simulink model "ECS_FOS"  (R2013b)
settings: Solver=ode45  StartTime=0.0  StopTime=10.0  RelTol=1e-3
values from neighbouring files (symbols this model uses):
  FuelBurn = [0 0 0 0 0 0 0 0 0 0 0 0 ... (18249 elements, 1x18249)]    [Benchmark_data1.mat]
undefined symbols (not defined in the file or in its folder): F1, F2, HUGHES_TREITLER, PN_70147
libraries: PowerFlowLib x47, simulink x6
(part 2 of 2)

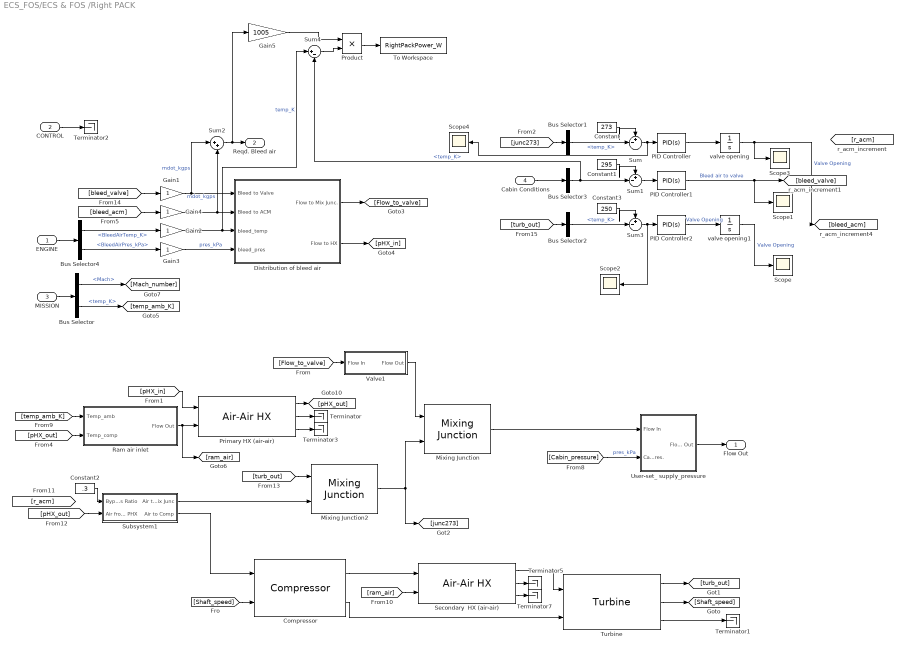
== system ECS_FOS/ECS & FOS /Right PACK ==
  ENGINE : Inport
  CONTROL : Inport  Port=2
  MISSION : Inport  Port=3
  Cabin Conditions : Inport  Port=4
  Bus Selector : BusSelector  OutputSignals=Flight parameters.Mach,Flight parameters.temp_K
  Bus Selector1 : BusSelector  OutputSignals=temp_K
  Bus Selector2 : BusSelector  OutputSignals=temp_K
  Bus Selector3 : BusSelector  OutputSignals=temp_K
  Bus Selector4 : BusSelector  OutputSignals=Bleed.BleedAirTemp_K,Bleed.BleedAirPres_kPa
  Compressor : PowerFlowLib/Energy & Power Systems/Thermal/ECS/Compressor
  Constant : Constant  Value=273
  Constant1 : Constant  Value=295
  Constant2 : Constant  Value=.3
  Constant3 : Constant  Value=250
  Distribution of bleed air : Subsystem
      mask Display:
      | port_label('input',1,'{ \bfBleed air to valve [kg/s]}','texmode','on')
      | port_label('input',2,'{ \bfBleed air to ACM [kg/s]}','texmode','on')
      | port_label('input',3,'{ \bfBleed temp. (K)}','texmode','on');
      | port_label('input',4,'{ \bfBleed pressure. (kPa)}','texmode','on')
      | 
      | 
      | 
      | port_label('output',1,'{\bfFlow to Mix Junc. }','texmode','on')
      | port_label('output',2,'{\bfFlow to ACM }','texmode','on')
  Gain{1..4} (4 alike) : Gain
  Gain5 : Gain  Gain=1005
  Mixing Junction : PowerFlowLib/Energy & Power Systems/Thermal/ECS/Mixing Junction  d_in_1=0.1  d_in_2=0.1  d_out=0.2
  Mixing Junction2 : PowerFlowLib/Energy & Power Systems/Thermal/ECS/Mixing Junction  d_in_1=0.1  d_in_2=0.1  d_out=0.2
  PID Controller : simulink/Continuous/PID Controller  Controller=PID  TimeDomain=Continuous-time  SampleTime=1  IntegratorMethod=Forward Euler  FilterMethod=Forward Euler  Form=Parallel  P=.01  I=0  D=0  N=100  InitialConditionSource=internal  InitialConditionForIntegrator=0  InitialConditionForFilter=0  ExternalReset=none  LimitOutput=off  UpperSaturationLimit=inf  LowerSaturationLimit=-inf  LinearizeAsGain=off  AntiWindupMode=none  Kb=1  TrackingMode=off  Kt=1  PParamMin=[]  PParamMax=[]  IParamMin=[]  IParamMax=[]  DParamMin=[]  DParamMax=[]  NParamMin=[]  NParamMax=[]  KbParamMin=[]  KbParamMax=[]  KtParamMin=[]  KtParamMax=[]  POutMin=[]  POutMax=[]  IOutMin=[]  IOutMax=[]  DOutMin=[]  DOutMax=[]  NOutMin=[]  NOutMax=[]  KbOutMin=[]  KbOutMax=[]  KtOutMin=[]  KtOutMax=[]  IntegratorOutMin=[]  IntegratorOutMax=[]  FilterOutMin=[]  FilterOutMax=[]  SumOutMin=[]  SumOutMax=[]  SumI1OutMin=[]  SumI1OutMax=[]  SumI2OutMin=[]  SumI2OutMax=[]  SumI3OutMin=[]  SumI3OutMax=[]  SumDOutMin=[]  SumDOutMax=[]  SaturationOutMin=[]  SaturationOutMax=[]  IntegratorContinuousStateAttributes=''  IntegratorStateMustResolveToSignalObject=off  IntegratorRTWStateStorageClass=Auto  FilterContinuousStateAttributes=''  FilterStateMustResolveToSignalObject=off  FilterRTWStateStorageClass=Auto
  PID Controller1 : simulink/Continuous/PID Controller  Controller=PID  TimeDomain=Continuous-time  SampleTime=1  IntegratorMethod=Forward Euler  FilterMethod=Forward Euler  Form=Parallel  P=.2  I=.01  D=0  N=100  InitialConditionSource=internal  InitialConditionForIntegrator=0  InitialConditionForFilter=0  ExternalReset=none  LimitOutput=on  UpperSaturationLimit=2  LowerSaturationLimit=.05  LinearizeAsGain=off  AntiWindupMode=none  Kb=1  TrackingMode=off  Kt=1  PParamMin=[]  PParamMax=[]  IParamMin=[]  IParamMax=[]  DParamMin=[]  DParamMax=[]  NParamMin=[]  NParamMax=[]  KbParamMin=[]  KbParamMax=[]  KtParamMin=[]  KtParamMax=[]  POutMin=[]  POutMax=[]  IOutMin=[]  IOutMax=[]  DOutMin=[]  DOutMax=[]  NOutMin=[]  NOutMax=[]  KbOutMin=[]  KbOutMax=[]  KtOutMin=[]  KtOutMax=[]  IntegratorOutMin=[]  IntegratorOutMax=[]  FilterOutMin=[]  FilterOutMax=[]  SumOutMin=[]  SumOutMax=[]  SumI1OutMin=[]  SumI1OutMax=[]  SumI2OutMin=[]  SumI2OutMax=[]  SumI3OutMin=[]  SumI3OutMax=[]  SumDOutMin=[]  SumDOutMax=[]  SaturationOutMin=[]  SaturationOutMax=[]  IntegratorContinuousStateAttributes=''  IntegratorStateMustResolveToSignalObject=off  IntegratorRTWStateStorageClass=Auto  FilterContinuousStateAttributes=''  FilterStateMustResolveToSignalObject=off  FilterRTWStateStorageClass=Auto
  PID Controller2 : simulink/Continuous/PID Controller  Controller=PID  TimeDomain=Continuous-time  SampleTime=1  IntegratorMethod=Forward Euler  FilterMethod=Forward Euler  Form=Parallel  P=0.01  I=0  D=0  N=100  InitialConditionSource=internal  InitialConditionForIntegrator=0  InitialConditionForFilter=0  ExternalReset=none  LimitOutput=off  UpperSaturationLimit=inf  LowerSaturationLimit=0  LinearizeAsGain=off  AntiWindupMode=none  Kb=1  TrackingMode=off  Kt=1  PParamMin=[]  PParamMax=[]  IParamMin=[]  IParamMax=[]  DParamMin=[]  DParamMax=[]  NParamMin=[]  NParamMax=[]  KbParamMin=[]  KbParamMax=[]  KtParamMin=[]  KtParamMax=[]  POutMin=[]  POutMax=[]  IOutMin=[]  IOutMax=[]  DOutMin=[]  DOutMax=[]  NOutMin=[]  NOutMax=[]  KbOutMin=[]  KbOutMax=[]  KtOutMin=[]  KtOutMax=[]  IntegratorOutMin=[]  IntegratorOutMax=[]  FilterOutMin=[]  FilterOutMax=[]  SumOutMin=[]  SumOutMax=[]  SumI1OutMin=[]  SumI1OutMax=[]  SumI2OutMin=[]  SumI2OutMax=[]  SumI3OutMin=[]  SumI3OutMax=[]  SumDOutMin=[]  SumDOutMax=[]  SaturationOutMin=[]  SaturationOutMax=[]  IntegratorContinuousStateAttributes=''  IntegratorStateMustResolveToSignalObject=off  IntegratorRTWStateStorageClass=Auto  FilterContinuousStateAttributes=''  FilterStateMustResolveToSignalObject=off  FilterRTWStateStorageClass=Auto
  Primary HX (air-air) : PowerFlowLib/Energy & Power Systems/Thermal/ECS/Air-Air HX  L_hx=0.2  W_hx=0.2  H_hx=0.2  t_p=0.0008  K_p=167  cp_hx=883  m_cm=16  l_fin=.005  t_fin=0.0002  s_fin=0.0015  h_fin=0.0095  K_n=167  eta_f=0.8  T_cm_0=50
  Product : Product
  Ram air inlet : Subsystem  mask{ram_air=.5, T_35=273}
      mask prompts: ram_air "Ram air mass flow rate"; T_35 "Temperature control for 35F valve"
      mask Display:
      | port_label('input',1,'{ \bf Ambient Temp.}','texmode','on')
      | port_label('input',2,'{ \bf Comp. Face Temp.}','texmode','on');
      | 
      | port_label('output',1,'{\bf Flow Out}','texmode','on')
  Scope{,1..4} (5 alike) : Scope
      Scope settings: SaveName=ScopeData32  SampleInput=on  SampleTime=1
      Scope1 settings: YMin=0  YMax=0.375  SaveName=ScopeData33  SampleInput=on  SampleTime=1
      Scope2 settings: YMin=-0.07  YMax=-0.0325  SaveName=ScopeData34  SampleInput=on  SampleTime=1
      Scope3 settings: YMin=0.427  YMax=0.437  SaveName=ScopeData35  SampleInput=on  SampleTime=1
      Scope4 settings: YMin=0.048825  YMax=0.04905  SaveName=ScopeData37  SampleInput=on  SampleTime=1
  Secondary  HX (air-air) : PowerFlowLib/Energy & Power Systems/Thermal/ECS/Air-Air HX  L_hx=0.2  W_hx=0.2  H_hx=0.2  t_p=0.0008  K_p=167  cp_hx=883  m_cm=16  l_fin=.005  t_fin=0.0002  s_fin=0.0015  h_fin=0.0095  K_n=167  eta_f=0.8  T_cm_0=25
  Subsystem1 : Subsystem
  Sum : Sum  Inputs=+-|
  Sum1 : Sum  Inputs=+-|
  Sum2 : Sum  Inputs=|++
  Sum3 : Sum  Inputs=+-|
  Sum4 : Sum  Inputs=|+-
  Terminator{,1..3,5,7} (6 alike) : Terminator
  To Workspace : ToWorkspace  VariableName=RightPackPower_W  SampleTime=10  SaveFormat=Structure With Time
  Turbine : PowerFlowLib/Energy & Power Systems/Thermal/ECS/Turbine  press_Turbine_exit=80  inertia=5e-5  n_t=0.7
  User-set_ supply_pressure : Subsystem
  Valve1 : Subsystem
  valve opening : Integrator  InitialCondition=.5  LimitOutput=on  UpperSaturationLimit=0.8  LowerSaturationLimit=0.2
  valve opening1 : Integrator  InitialCondition=.5  LimitOutput=on  UpperSaturationLimit=1  LowerSaturationLimit=.3
  Flow Out : Outport
  Reqd. Bleed air : Outport  Port=2
  wires:
  Product/1 -> To Workspace/1
  Sum4/1 -> Product/2
  Gain5/1 -> Product/1
  Sum2/1 -> Reqd. Bleed air/1, Gain5/1
  Gain2/1 -> Distribution of bleed air/3(bleed_temp), Sum4/1  "temp_K"
  Bus Selector3/1 -> Sum1/2, Sum4/2  "<temp_K>"
  Constant2/1 -> Subsystem1/1(Bypass Ratio)
  [bleed_acm] -> Gain4/1
  Constant1/1 -> Sum1/1
  PID Controller1/1 -> [bleed_valve], Scope1/1  "Bleed air to valve"
  Sum1/1 -> PID Controller1/1
  [pHX_in] -> Primary HX (air-air)/1
  Valve1/1(Flow Out) -> Mixing Junction/1
  [Flow_to_valve] -> Valve1/1(Flow In)
  [Shaft_speed] -> Compressor/2
  Compressor/2 -> Turbine/2
  Ram air inlet/1(Flow Out) -> Primary HX (air-air)/2, [ram_air]
  Compressor/1 -> Secondary  HX (air-air)/1
  [ram_air] -> Secondary  HX (air-air)/2
  Mixing Junction/1 -> User-set_ supply_pressure/1(Flow In)
  Turbine/2 -> [Shaft_speed]
  Turbine/3 -> Terminator1/1
  Turbine/1 -> [turb_out]
  User-set_ supply_pressure/1(Flow Out) -> Flow Out/1
  [Cabin_pressure] -> User-set_ supply_pressure/2(Cabin Pres.)  "pres_kPa"
  [temp_amb_K] -> Ram air inlet/1(Temp_amb)
  [pHX_out] -> Ram air inlet/2(Temp_comp)
  MISSION/1 -> Bus Selector/1
  CONTROL/1 -> Terminator2/1
  ENGINE/1 -> Bus Selector4/1
  Distribution of bleed air/2(Flow to HX) -> [pHX_in]
  Distribution of bleed air/1(Flow to Mix Junc.) -> [Flow_to_valve]
  Bus Selector4/1 -> Gain2/1  "<BleedAirTemp_K>"
  Bus Selector4/2 -> Gain3/1  "<BleedAirPres_kPa>"
  Bus Selector/2 -> [temp_amb_K]  "<temp_K>"
  Bus Selector/1 -> [Mach_number]  "<Mach>"
  Gain1/1 -> Distribution of bleed air/1(Bleed to Valve), Sum2/1  "mdot_kgps"
  Gain3/1 -> Distribution of bleed air/4(bleed_pres)  "pres_kPa"
  [bleed_valve] -> Gain1/1
  Primary HX (air-air)/3 -> Terminator3/1
  Primary HX (air-air)/2 -> Terminator/1
  Primary HX (air-air)/1 -> [pHX_out]
  Secondary  HX (air-air)/2 -> Terminator5/1
  Secondary  HX (air-air)/3 -> Terminator7/1
  Secondary  HX (air-air)/1 -> Turbine/1
  [pHX_out] -> Subsystem1/2(Air from PHX)
  Mixing Junction2/1 -> [junc273], Mixing Junction/2
  [turb_out] -> Mixing Junction2/1
  Subsystem1/1(Air to Mix Junc) -> Mixing Junction2/2
  Subsystem1/2(Air to Comp) -> Compressor/1
  [junc273] -> Bus Selector1/1
  Bus Selector1/1 -> Sum/2  "<temp_K>"
  Sum/1 -> PID Controller/1, Scope4/1
  PID Controller/1 -> valve opening/1
  valve opening/1 -> [bleed_acm], Scope3/1  "Valve Opening"
  Constant/1 -> Sum/1
  Gain4/1 -> Distribution of bleed air/2(Bleed to ACM), Sum2/2  "mdot_kgps"
  [turb_out] -> Bus Selector2/1
  Bus Selector2/1 -> Sum3/2  "<temp_K>"
  Sum3/1 -> PID Controller2/1, Scope2/1
  PID Controller2/1 -> valve opening1/1  "Valve Opening"
  Constant3/1 -> Sum3/1
  valve opening1/1 -> Scope/1  "Valve Opening"
  Cabin Conditions/1 -> Bus Selector3/1

== system ECS_FOS/ECS & FOS /Thermal_sources_from Electrical_power_model1 ==
  Gain : Gain
  Terminator : Terminator
  Terminator1 : Terminator
  Terminator2 : Terminator
  ThermalSource : Subsystem  Tag=Flow  Description=TwoPhase  mask(Thermal Source){load_loc=Cockpit}
      mask prompts: load_loc "Location"
      mask help: Output of all thermal loads from the selected location. Loads are in Watts.
      mask init:
      | init_thermal_sourcesink(1)
      settings: CopyFcn=|
      | vals = get_param(gcb,'MaskValues');
      | set_param(gcb,'MaskValues',[vals(1);num2str(0)]);
      mask TypeOptions load_loc: Cockpit | Cabin | CargoBay | LeftWing | RightWing | Empennage
      mask Display:
      | text(.5,.7,'Thermal Source','horizontalAlignment','center','texmode','on')
      | text(.5,.4,get_param(gcb,'load_loc'),'horizontalAlignment','center','texmode','on')
  ThermalSource3 : Subsystem  Tag=Flow  Description=TwoPhase  mask(Thermal Source){load_loc=RightWing}
      mask prompts: load_loc "Location"
      mask help: Output of all thermal loads from the selected location. Loads are in Watts.
      mask init:
      | init_thermal_sourcesink(1)
      settings: CopyFcn=|
      | vals = get_param(gcb,'MaskValues');
      | set_param(gcb,'MaskValues',[vals(1);num2str(0)]);
      mask TypeOptions load_loc: Cockpit | Cabin | CargoBay | LeftWing | RightWing | Empennage
      mask Display:
      | text(.5,.7,'Thermal Source','horizontalAlignment','center','texmode','on')
      | text(.5,.4,get_param(gcb,'load_loc'),'horizontalAlignment','center','texmode','on')
  ThermalSource4 : Subsystem  Tag=Flow  Description=TwoPhase  mask(Thermal Source){load_loc=Empennage}
      mask prompts: load_loc "Location"
      mask help: Output of all thermal loads from the selected location. Loads are in Watts.
      mask init:
      | init_thermal_sourcesink(1)
      settings: CopyFcn=|
      | vals = get_param(gcb,'MaskValues');
      | set_param(gcb,'MaskValues',[vals(1);num2str(0)]);
      mask TypeOptions load_loc: Cockpit | Cabin | CargoBay | LeftWing | RightWing | Empennage
      mask Display:
      | text(.5,.7,'Thermal Source','horizontalAlignment','center','texmode','on')
      | text(.5,.4,get_param(gcb,'load_loc'),'horizontalAlignment','center','texmode','on')
  ThermalSource5 : Subsystem  Tag=Flow  Description=TwoPhase  mask(Thermal Source){load_loc=LeftWing}
      mask prompts: load_loc "Location"
      mask help: Output of all thermal loads from the selected location. Loads are in Watts.
      mask init:
      | init_thermal_sourcesink(1)
      settings: CopyFcn=|
      | vals = get_param(gcb,'MaskValues');
      | set_param(gcb,'MaskValues',[vals(1);num2str(0)]);
      mask TypeOptions load_loc: Cockpit | Cabin | CargoBay | LeftWing | RightWing | Empennage
      mask Display:
      | text(.5,.7,'Thermal Source','horizontalAlignment','center','texmode','on')
      | text(.5,.4,get_param(gcb,'load_loc'),'horizontalAlignment','center','texmode','on')
  Thermal Loads : Outport
  wires:
  ThermalSource5/1(Load) -> Terminator/1
  ThermalSource4/1(Load) -> Terminator2/1
  ThermalSource3/1(Load) -> Terminator1/1
  Gain/1 -> Thermal Loads/1
  ThermalSource/1(Load) -> Gain/1

== system ECS_FOS/Engine #1 - updated 12//1/Heat Loads ==
  Flow In : Inport
  Bus Creator : BusCreator
  Bus Selector : BusSelector  OutputSignals=temp_K,mdot_kgps,pres_kPa,h_kJ/kg
  Gain : Gain  Gain=.1
  Random Number : RandomNumber  Mean=20  Variance=10  SampleTime=0.1
  Sum : Sum  Inputs=++|
  Flow Out : Outport
  wires:
  Flow In/1 -> Bus Selector/1
  Bus Selector/1 -> Sum/2  "<temp_K>"
  Random Number/1 -> Sum/1
  Bus Creator/1 -> Flow Out/1
  Sum/1 -> Bus Creator/1  "temp_K"
  Bus Selector/2 -> Bus Creator/2  "<mdot_kgps>"
  Bus Selector/3 -> Gain/1  "<pres_kPa>"
  Bus Selector/4 -> Bus Creator/4  "<h_kJ/kg>"
  Gain/1 -> Bus Creator/3  "pres_kPa"

== system ECS_FOS/Engine #1 - updated 12//10/Heat Loads ==
  Flow In : Inport
  Bus Creator : BusCreator
  Bus Selector : BusSelector  OutputSignals=temp_K,mdot_kgps,pres_kPa,h_kJ/kg
  Gain : Gain  Gain=.1
  Random Number : RandomNumber  Mean=20  Variance=10  SampleTime=0.1
  Sum : Sum  Inputs=++|
  Flow Out : Outport
  wires:
  Gain/1 -> Bus Creator/3  "pres_kPa"
  Bus Selector/4 -> Bus Creator/4  "<h_kJ/kg>"
  Bus Selector/3 -> Gain/1  "<pres_kPa>"
  Bus Selector/2 -> Bus Creator/2  "<mdot_kgps>"
  Sum/1 -> Bus Creator/1  "temp_K"
  Bus Creator/1 -> Flow Out/1
  Random Number/1 -> Sum/1
  Bus Selector/1 -> Sum/2  "<temp_K>"
  Flow In/1 -> Bus Selector/1

== system ECS_FOS/ECS & FOS /FOHX Left Wing/HX_Calcs ==
  Inputs : Inport
  Bus Creator1 : BusCreator
  Bus Creator2 : BusCreator  Inputs=2
  Fluid 1 Heat Transfer Calculation : Subsystem  TreatAsAtomicUnit=on
  Fluid 2 Heat Transfer Calculation : Subsystem  TreatAsAtomicUnit=on
  Input Processing : Subsystem
  Out : Outport
  wires:
  Fluid 1 Heat Transfer Calculation/3(q_h) -> [q1]
  Fluid 1 Heat Transfer Calculation/2(T_out_h) -> [T1_out]
  Fluid 1 Heat Transfer Calculation/1(h_out_h) -> [h1_out]
  Bus Creator1/1 -> Out/1  "Outputs"
  [Inputs] -> Fluid 1 Heat Transfer Calculation/1(Inputs)
  Inputs/1 -> Input Processing/1(Inputs)  "Inputs"
  Input Processing/1(Processed_Inputs) -> [Inputs]
  Fluid 2 Heat Transfer Calculation/3(q_h) -> [q2]
  Fluid 2 Heat Transfer Calculation/2(T_out) -> [T2_out]
  Fluid 2 Heat Transfer Calculation/1(h_out) -> [h2_out]
  [Inputs] -> Fluid 2 Heat Transfer Calculation/1(Inputs)
  [q1] -> Bus Creator2/1
  [q2] -> Bus Creator2/2
  Bus Creator2/1 -> [q]
  [T2_out] -> Bus Creator1/4  "T2_out"
  [h1_out] -> Bus Creator1/1  "h1_out"
  [T1_out] -> Bus Creator1/2  "T1_out"
  [h2_out] -> Bus Creator1/3  "h2_out"

== system ECS_FOS/ECS & FOS /FOHX Right Wing/HX_Calcs ==
  Inputs : Inport
  Bus Creator1 : BusCreator
  Bus Creator2 : BusCreator  Inputs=2
  Fluid 1 Heat Transfer Calculation : Subsystem  TreatAsAtomicUnit=on
  Fluid 2 Heat Transfer Calculation : Subsystem  TreatAsAtomicUnit=on
  Input Processing : Subsystem
  Out : Outport
  wires:
  [h2_out] -> Bus Creator1/3  "h2_out"
  [T1_out] -> Bus Creator1/2  "T1_out"
  [h1_out] -> Bus Creator1/1  "h1_out"
  [T2_out] -> Bus Creator1/4  "T2_out"
  Bus Creator2/1 -> [q]
  [q2] -> Bus Creator2/2
  [q1] -> Bus Creator2/1
  [Inputs] -> Fluid 2 Heat Transfer Calculation/1(Inputs)
  Fluid 2 Heat Transfer Calculation/1(h_out) -> [h2_out]
  Fluid 2 Heat Transfer Calculation/2(T_out) -> [T2_out]
  Fluid 2 Heat Transfer Calculation/3(q_h) -> [q2]
  Input Processing/1(Processed_Inputs) -> [Inputs]
  Inputs/1 -> Input Processing/1(Inputs)  "Inputs"
  [Inputs] -> Fluid 1 Heat Transfer Calculation/1(Inputs)
  Bus Creator1/1 -> Out/1  "Outputs"
  Fluid 1 Heat Transfer Calculation/1(h_out_h) -> [h1_out]
  Fluid 1 Heat Transfer Calculation/2(T_out_h) -> [T1_out]
  Fluid 1 Heat Transfer Calculation/3(q_h) -> [q1]

== system ECS_FOS/ECS & FOS /Fuel Tanks//Pumps/FlowGenerator1 ==
  Bias : Bias  Bias=273.15
  Bus Creator1 : BusCreator
  Constant3 : Constant  Value=flowenthalpy
  Constant5 : Constant  Value=flowrate
  Constant6 : Constant  Value=flowtemp
  Constant7 : Constant  Value=flowpres
  FlowOut : Outport  Tag=Flow Out
  wires:
  Bus Creator1/1 -> FlowOut/1  "Outlet"
  Constant6/1 -> Bias/1  "temp_C"
  Constant7/1 -> Bus Creator1/3  "pres_kPa"
  Constant3/1 -> Bus Creator1/4  "H_kJpkg"
  Constant5/1 -> Bus Creator1/1  "mdot_kgps"
  Bias/1 -> Bus Creator1/2  "temp_K"

== system ECS_FOS/ECS & FOS /Fuel Tanks//Pumps/Fuel Control Left Wing ==
  FuelNeed : Inport
  FuelFromPump : Inport  Port=2
  Bus Creator : BusCreator  Inputs=3
  Bus Creator1 : BusCreator  Inputs=3
  Bus Selector : BusSelector  OutputSignals=mdot_kgps,temp_K,pres_kPa
  Gain : Gain
  Gain1 : Gain
  Saturation : Saturate  UpperLimit=inf  LowerLimit=0
  Sum : Sum  Inputs=|+-
  Switch : Switch  Criteria=u2 > Threshold
  Fuel2Engine : Outport
  Fuel2Tank : Outport  Port=2
  wires:
  FuelFromPump/1 -> Bus Selector/1
  Bus Selector/1 -> Sum/1, Switch/3  "<mdot_kgps>"
  FuelNeed/1 -> Sum/2, Switch/1
  Sum/1 -> Saturation/1, Switch/2
  Bus Creator/1 -> Fuel2Tank/1
  Bus Selector/2 -> Bus Creator/2, Gain1/1  "<temp_K>"
  Saturation/1 -> Bus Creator/1  "mdot_kgps"
  Switch/1 -> Bus Creator1/1  "mdot_kgps"
  Bus Selector/3 -> Bus Creator/3, Gain/1  "<pres_kPa>"
  Bus Creator1/1 -> Fuel2Engine/1
  Gain/1 -> Bus Creator1/3  "pres_kPa"
  Gain1/1 -> Bus Creator1/2  "temp_K"

== system ECS_FOS/ECS & FOS /Fuel Tanks//Pumps/Fuel Control Right Wing  ==
  FuelNeed : Inport
  FuelFromPump : Inport  Port=2
  Bus Creator : BusCreator  Inputs=3
  Bus Creator1 : BusCreator  Inputs=3
  Bus Selector : BusSelector  OutputSignals=mdot_kgps,temp_K,pres_kPa
  Gain : Gain
  Gain1 : Gain
  Saturation : Saturate  UpperLimit=inf  LowerLimit=0
  Sum : Sum  Inputs=|+-
  Switch : Switch  Criteria=u2 > Threshold
  Fuel2Engine : Outport
  Fuel2Tank : Outport  Port=2
  wires:
  Gain1/1 -> Bus Creator1/2  "temp_K"
  Gain/1 -> Bus Creator1/3  "pres_kPa"
  Bus Creator1/1 -> Fuel2Engine/1
  Bus Selector/3 -> Gain/1, Bus Creator/3  "<pres_kPa>"
  Switch/1 -> Bus Creator1/1  "mdot_kgps"
  Saturation/1 -> Bus Creator/1  "mdot_kgps"
  Bus Selector/2 -> Gain1/1, Bus Creator/2  "<temp_K>"
  Bus Creator/1 -> Fuel2Tank/1
  Sum/1 -> Switch/2, Saturation/1
  FuelNeed/1 -> Switch/1, Sum/2
  Bus Selector/1 -> Switch/3, Sum/1  "<mdot_kgps>"
  FuelFromPump/1 -> Bus Selector/1

== system ECS_FOS/ECS & FOS /Fuel Tanks//Pumps/Fuel Switch On//Off ==
  Right Wing Tank : Inport
  Center Tank : Inport  Port=2
  Left Wing Tank : Inport  Port=3
  Operating RPM : Constant  Value=6000
  Operating RPM1 : Constant  Value=6000
  Operating RPM2 : Constant  Value=6000
  Right Wing Fuel Pumps On/Off : Switch  Criteria=u2 ~= 0
  Right Wing Fuel Pumps On/Off1 : Switch  Criteria=u2 ~= 0
  Right Wing Fuel Pumps On/Off2 : Switch  Criteria=u2 ~= 0
  shut off : Constant  Value=0
  shut off1 : Constant  Value=0
  shut off2 : Constant  Value=0
  Right Wing RPM : Outport
  Left Wing RPM : Outport  Port=2
  Center RPM : Outport  Port=3
  wires:
  Right Wing Fuel Pumps On/Off2/1 -> Left Wing RPM/1
  Right Wing Fuel Pumps On/Off1/1 -> Center RPM/1
  Right Wing Fuel Pumps On/Off/1 -> Right Wing RPM/1
  Left Wing Tank/1 -> Right Wing Fuel Pumps On/Off2/2
  shut off2/1 -> Right Wing Fuel Pumps On/Off2/3
  Operating RPM2/1 -> Right Wing Fuel Pumps On/Off2/1
  Center Tank/1 -> Right Wing Fuel Pumps On/Off1/2
  shut off1/1 -> Right Wing Fuel Pumps On/Off1/3
  Operating RPM1/1 -> Right Wing Fuel Pumps On/Off1/1
  Right Wing Tank/1 -> Right Wing Fuel Pumps On/Off/2
  shut off/1 -> Right Wing Fuel Pumps On/Off/3
  Operating RPM/1 -> Right Wing Fuel Pumps On/Off/1

== system ECS_FOS/ECS & FOS /Fuel Tanks//Pumps/Pump Split ==
  Flow In : Inport
  Bus Creator : BusCreator
  Bus Selector14 : BusSelector  OutputSignals=temp_K,mdot_kgps,pres_kPa,H_kJpkg
  Gain : Gain  Gain=0.5
  Flow Out : Outport
  wires:
  Flow In/1 -> Bus Selector14/1
  Bus Selector14/2 -> Gain/1  "<mdot_kgps>"
  Bus Creator/1 -> Flow Out/1
  Bus Selector14/1 -> Bus Creator/1  "<temp_K>"
  Gain/1 -> Bus Creator/2  "mdot_kgps"
  Bus Selector14/3 -> Bus Creator/3  "<pres_kPa>"
  Bus Selector14/4 -> Bus Creator/4  "<H_kJpkg>"

== system ECS_FOS/ECS & FOS /Fuel Tanks//Pumps/Pump Split1 ==
  Flow In : Inport
  Bus Creator : BusCreator
  Bus Selector14 : BusSelector  OutputSignals=temp_K,mdot_kgps,pres_kPa,H_kJpkg
  Gain : Gain  Gain=0.5
  Flow Out : Outport
  wires:
  Bus Selector14/4 -> Bus Creator/4  "<H_kJpkg>"
  Bus Selector14/3 -> Bus Creator/3  "<pres_kPa>"
  Gain/1 -> Bus Creator/2  "mdot_kgps"
  Bus Selector14/1 -> Bus Creator/1  "<temp_K>"
  Bus Creator/1 -> Flow Out/1
  Bus Selector14/2 -> Gain/1  "<mdot_kgps>"
  Flow In/1 -> Bus Selector14/1

== system ECS_FOS/ECS & FOS /Fuel Tanks//Pumps/Pump Split2 ==
  Flow In : Inport
  Bus Creator : BusCreator
  Bus Selector14 : BusSelector  OutputSignals=temp_K,mdot_kgps,pres_kPa,H_kJpkg
  Gain : Gain  Gain=0.5
  Flow Out : Outport
  wires:
  Bus Selector14/4 -> Bus Creator/4  "<H_kJpkg>"
  Bus Selector14/3 -> Bus Creator/3  "<pres_kPa>"
  Gain/1 -> Bus Creator/2  "mdot_kgps"
  Bus Selector14/1 -> Bus Creator/1  "<temp_K>"
  Bus Creator/1 -> Flow Out/1
  Bus Selector14/2 -> Gain/1  "<mdot_kgps>"
  Flow In/1 -> Bus Selector14/1

== system ECS_FOS/ECS & FOS /Left PACK/Distribution of bleed air ==
  Bleed to Valve : Inport
  Bleed to ACM : Inport  Port=2
  bleed_temp : Inport  Port=3
  bleed_pres : Inport  Port=4
  Bus Creator1 : BusCreator  Inputs=3
  Bus Creator2 : BusCreator  Inputs=3
  Scope : Scope  NumInputPorts=4
      settings: YMin=0~386.7~110~0.2  YMax=0.055~387.8~160~0.85  SaveName=ScopeData42  SampleInput=on  SampleTime=1
  Flow to Mix Junc. : Outport
  Flow to HX : Outport  Port=2
  wires:
  Bus Creator2/1 -> Flow to HX/1
  Bus Creator1/1 -> Flow to Mix Junc./1
  Bleed to Valve/1 -> Scope/1, Bus Creator1/1  "mdot_kgps"
  bleed_pres/1 -> Scope/3, Bus Creator1/3, Bus Creator2/3
  bleed_temp/1 -> Scope/2, Bus Creator1/2, Bus Creator2/2
  Bleed to ACM/1 -> Scope/4, Bus Creator2/1  "mdot_kgps"

== system ECS_FOS/ECS & FOS /Left PACK/Ram air inlet ==
  Temp_amb : Inport
  Temp_comp : Inport  Port=2
  2 : Constant  Value=T_35
  Bus Creator : BusCreator  Inputs=3
  Bus Selector4 : BusSelector  OutputSignals=temp_K
  Constant1 : Constant  Value=22.5
  Gain : Gain  Gain=0.95
  Gain1 : Gain
  Memory : Memory  X0=ram_air
  Subtract : Sum  Inputs=+-
  Switch : Switch  Criteria=u2 ~= 0  Threshold=30
  Flow Out : Outport
  wires:
  Gain1/1 -> Switch/1
  Memory/1 -> Gain/1, Gain1/1, Bus Creator/3  "mdot_kgps"
  Bus Creator/1 -> Flow Out/1
  Constant1/1 -> Bus Creator/2  "pres_kPa"
  Temp_amb/1 -> Bus Creator/1  "temp_K"
  Switch/1 -> Memory/1
  Gain/1 -> Switch/3
  Subtract/1 -> Switch/2
  2/1 -> Subtract/2
  Bus Selector4/1 -> Subtract/1  "<temp_K>"
  Temp_comp/1 -> Bus Selector4/1

== system ECS_FOS/ECS & FOS /Left PACK/Subsystem1 ==
  Bypass Ratio : Inport
  Air from PHX : Inport  Port=2
  Bus Creator : BusCreator  Inputs=3
  Bus Creator1 : BusCreator  Inputs=3
  Bus Selector : BusSelector  OutputSignals=mdot_kgps,temp_K,pres_kPa
  Fcn1 : Fcn  Expr=1-u(1)
  Gain : Gain
  Gain1 : Gain
  Gain2 : Gain
  Product : Product  RndMeth=Zero
  Product1 : Product  RndMeth=Zero
  Saturation : Saturate  UpperLimit=inf  LowerLimit=eps
  Air to Mix Junc : Outport
  Air to Comp : Outport  Port=2
  wires:
  Gain2/1 -> Bus Creator/3  "pres_kPa"
  Fcn1/1 -> Product/1
  Bypass Ratio/1 -> Product1/2, Fcn1/1
  Product/1 -> Saturation/1
  Air from PHX/1 -> Bus Selector/1
  Bus Selector/1 -> Product1/1, Product/2  "<mdot_kgps>"
  Bus Creator/1 -> Air to Comp/1
  Bus Selector/2 -> Bus Creator/2, Gain1/1  "<temp_K>"
  Saturation/1 -> Bus Creator/1  "mdot_kgps"
  Product1/1 -> Bus Creator1/1  "mdot_kgps"
  Bus Selector/3 -> Gain2/1, Gain/1  "<pres_kPa>"
  Bus Creator1/1 -> Air to Mix Junc/1
  Gain/1 -> Bus Creator1/3  "pres_kPa"
  Gain1/1 -> Bus Creator1/2  "temp_K"

== system ECS_FOS/ECS & FOS /Left PACK/User-set_ supply_pressure ==
  Flow In : Inport
  Cabin Pres. : Inport  Port=2
  Bus Creator4 : BusCreator  Inputs=3
  Bus Selector3 : BusSelector  OutputSignals=mdot_kgps,temp_K
  Gain1 : Gain  Gain=1.1
  Flow Out : Outport
  wires:
  Cabin Pres./1 -> Gain1/1
  Bus Creator4/1 -> Flow Out/1
  Flow In/1 -> Bus Selector3/1
  Gain1/1 -> Bus Creator4/3  "pres_kPa"
  Bus Selector3/2 -> Bus Creator4/2  "<temp_K>"
  Bus Selector3/1 -> Bus Creator4/1  "<mdot_kgps>"

== system ECS_FOS/ECS & FOS /Left PACK/Valve1 ==
  Flow In : Inport
  Bus Creator2 : BusCreator  Inputs=3
  Bus Selector2 : BusSelector  OutputSignals=mdot_kgps,pres_kPa,temp_K
  Math Functin : Math  Operator=pow  SaturateOnIntegerOverflow=on
  Product : Product  RndMeth=Zero
  Sum : Sum  Inputs=|-+
  "Value?? -- MAW" : Constant  Value=50
  get u : Gain
  mass_flow_rate1 : Constant  Value=2
  Flow Out : Outport
  wires:
  "Value?? -- MAW"/1 -> Product/1
  Bus Selector2/3 -> Bus Creator2/3  "<temp_K>"
  Sum/1 -> Bus Creator2/2  "pres_kPa"
  Bus Selector2/2 -> Sum/2  "<pres_kPa>"
  Product/1 -> Sum/1
  Math Functin/1 -> Product/2
  mass_flow_rate1/1 -> Math Functin/2
  get u/1 -> Math Functin/1
  Bus Selector2/1 -> get u/1, Bus Creator2/1  "<mdot_kgps>"
  Flow In/1 -> Bus Selector2/1
  Bus Creator2/1 -> Flow Out/1

== system ECS_FOS/ECS & FOS /Right PACK/Distribution of bleed air ==
  Bleed to Valve : Inport
  Bleed to ACM : Inport  Port=2
  bleed_temp : Inport  Port=3
  bleed_pres : Inport  Port=4
  Bus Creator1 : BusCreator  Inputs=3
  Bus Creator2 : BusCreator  Inputs=3
  Scope : Scope  NumInputPorts=4
      settings: YMin=0~386.7~110~0.2  YMax=0.055~387.8~160~0.85  SaveName=ScopeData42  SampleInput=on  SampleTime=1
  Flow to Mix Junc. : Outport
  Flow to HX : Outport  Port=2
  wires:
  Bleed to ACM/1 -> Bus Creator2/1, Scope/4  "mdot_kgps"
  bleed_temp/1 -> Bus Creator2/2, Bus Creator1/2, Scope/2
  bleed_pres/1 -> Bus Creator2/3, Bus Creator1/3, Scope/3
  Bleed to Valve/1 -> Bus Creator1/1, Scope/1  "mdot_kgps"
  Bus Creator1/1 -> Flow to Mix Junc./1
  Bus Creator2/1 -> Flow to HX/1

== system ECS_FOS/ECS & FOS /Right PACK/Ram air inlet ==
  Temp_amb : Inport
  Temp_comp : Inport  Port=2
  2 : Constant  Value=T_35
  Bus Creator : BusCreator  Inputs=3
  Bus Selector4 : BusSelector  OutputSignals=temp_K
  Constant1 : Constant  Value=22.5
  Gain : Gain  Gain=0.95
  Gain1 : Gain
  Memory : Memory  X0=ram_air
  Subtract : Sum  Inputs=+-
  Switch : Switch  Criteria=u2 ~= 0  Threshold=30
  Flow Out : Outport
  wires:
  Temp_comp/1 -> Bus Selector4/1
  Bus Selector4/1 -> Subtract/1  "<temp_K>"
  2/1 -> Subtract/2
  Subtract/1 -> Switch/2
  Gain/1 -> Switch/3
  Switch/1 -> Memory/1
  Temp_amb/1 -> Bus Creator/1  "temp_K"
  Constant1/1 -> Bus Creator/2  "pres_kPa"
  Bus Creator/1 -> Flow Out/1
  Memory/1 -> Bus Creator/3, Gain1/1, Gain/1  "mdot_kgps"
  Gain1/1 -> Switch/1

== system ECS_FOS/ECS & FOS /Right PACK/Subsystem1 ==
  Bypass Ratio : Inport
  Air from PHX : Inport  Port=2
  Bus Creator : BusCreator  Inputs=3
  Bus Creator1 : BusCreator  Inputs=3
  Bus Selector : BusSelector  OutputSignals=mdot_kgps,temp_K,pres_kPa
  Fcn1 : Fcn  Expr=1-u(1)
  Gain : Gain
  Gain1 : Gain
  Gain2 : Gain
  Product : Product  RndMeth=Zero
  Product1 : Product  RndMeth=Zero
  Saturation : Saturate  UpperLimit=inf  LowerLimit=eps
  Air to Mix Junc : Outport
  Air to Comp : Outport  Port=2
  wires:
  Gain1/1 -> Bus Creator1/2  "temp_K"
  Gain/1 -> Bus Creator1/3  "pres_kPa"
  Bus Creator1/1 -> Air to Mix Junc/1
  Bus Selector/3 -> Gain/1, Gain2/1  "<pres_kPa>"
  Product1/1 -> Bus Creator1/1  "mdot_kgps"
  Saturation/1 -> Bus Creator/1  "mdot_kgps"
  Bus Selector/2 -> Gain1/1, Bus Creator/2  "<temp_K>"
  Bus Creator/1 -> Air to Comp/1
  Bus Selector/1 -> Product/2, Product1/1  "<mdot_kgps>"
  Air from PHX/1 -> Bus Selector/1
  Product/1 -> Saturation/1
  Bypass Ratio/1 -> Fcn1/1, Product1/2
  Fcn1/1 -> Product/1
  Gain2/1 -> Bus Creator/3  "pres_kPa"

== system ECS_FOS/ECS & FOS /Right PACK/User-set_ supply_pressure ==
  Flow In : Inport
  Cabin Pres. : Inport  Port=2
  Bus Creator4 : BusCreator  Inputs=3
  Bus Selector3 : BusSelector  OutputSignals=mdot_kgps,temp_K
  Gain1 : Gain  Gain=1.1
  Flow Out : Outport
  wires:
  Bus Selector3/1 -> Bus Creator4/1  "<mdot_kgps>"
  Bus Selector3/2 -> Bus Creator4/2  "<temp_K>"
  Gain1/1 -> Bus Creator4/3  "pres_kPa"
  Flow In/1 -> Bus Selector3/1
  Bus Creator4/1 -> Flow Out/1
  Cabin Pres./1 -> Gain1/1

== system ECS_FOS/ECS & FOS /Right PACK/Valve1 ==
  Flow In : Inport
  Bus Creator2 : BusCreator  Inputs=3
  Bus Selector2 : BusSelector  OutputSignals=mdot_kgps,pres_kPa,temp_K
  Math Functin : Math  Operator=pow  SaturateOnIntegerOverflow=on
  Product : Product  RndMeth=Zero
  Sum : Sum  Inputs=|-+
  "Value?? -- MAW" : Constant  Value=50
  get u : Gain
  mass_flow_rate1 : Constant  Value=2
  Flow Out : Outport
  wires:
  Bus Creator2/1 -> Flow Out/1
  Flow In/1 -> Bus Selector2/1
  Bus Selector2/1 -> Bus Creator2/1, get u/1  "<mdot_kgps>"
  get u/1 -> Math Functin/1
  mass_flow_rate1/1 -> Math Functin/2
  Math Functin/1 -> Product/2
  Product/1 -> Sum/1
  Bus Selector2/2 -> Sum/2  "<pres_kPa>"
  Sum/1 -> Bus Creator2/2  "pres_kPa"
  Bus Selector2/3 -> Bus Creator2/3  "<temp_K>"
  "Value?? -- MAW"/1 -> Product/1

== system ECS_FOS/ECS & FOS /Thermal_sources_from Electrical_power_model1/ThermalSource ==
  LoadBus : BusCreator  Inputs=1
  Load : Outport
  wires:
  LoadBus/1 -> Load/1

== system ECS_FOS/ECS & FOS /Thermal_sources_from Electrical_power_model1/ThermalSource3 ==
  LoadBus : BusCreator  Inputs=1
  Load : Outport
  wires:
  LoadBus/1 -> Load/1

== system ECS_FOS/ECS & FOS /Thermal_sources_from Electrical_power_model1/ThermalSource4 ==
  LoadBus : BusCreator  Inputs=1
  Load : Outport
  wires:
  LoadBus/1 -> Load/1

== system ECS_FOS/ECS & FOS /Thermal_sources_from Electrical_power_model1/ThermalSource5 ==
  LoadBus : BusCreator  Inputs=1
  Load : Outport
  wires:
  LoadBus/1 -> Load/1

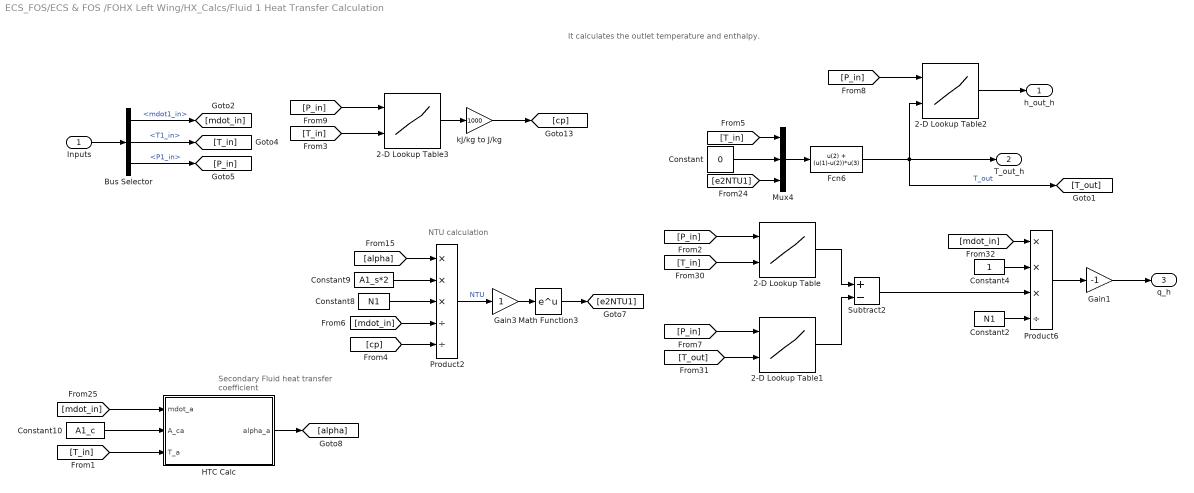
== system ECS_FOS/ECS & FOS /FOHX Left Wing/HX_Calcs/Fluid 1 Heat Transfer Calculation ==
  note: NTU calculation
  note: Secondary Fluid heat transfer coefficient
  note: It calculates the outlet temperature and enthalpy.
  Inputs : Inport
  2-D Lookup Table : Lookup_n-D  BreakpointsForDimension1=F1.P  BreakpointsForDimension2=F1.T  Table=F1.H_pt  RndMeth=Simplest  InputSameDT=on
  2-D Lookup Table1 : Lookup_n-D  BreakpointsForDimension1=F1.P  BreakpointsForDimension2=F1.T  Table=F1.H_pt  RndMeth=Simplest  InputSameDT=on
  2-D Lookup Table2 : Lookup_n-D  BreakpointsForDimension1=F1.P  BreakpointsForDimension2=F1.T  Table=F1.H_pt  RndMeth=Simplest  InputSameDT=on
  2-D Lookup Table3 : Lookup_n-D  BreakpointsForDimension1=F1.P  BreakpointsForDimension2=F1.T  Table=F1.Cp_pt  RndMeth=Simplest  InputSameDT=on
  Bus Selector : BusSelector  OutputSignals=mdot1_in,T1_in,P1_in
  Constant : Constant  Value=0
  Constant10 : Constant  Value=A1_c
  Constant2 : Constant  Value=N1
  Constant4 : Constant
  Constant8 : Constant  Value=N1
  Constant9 : Constant  Value=A1_s*2
  Fcn6 : Fcn  Expr=u(2) + (u(1)-u(2))*u(3)
  Gain1 : Gain  Gain=-1
  Gain3 : Gain
  HTC Calc : Subsystem
  Math Function3 : Math  SaturateOnIntegerOverflow=on
  Mux4 : Mux  Inputs=3
  Product2 : Product  Inputs=***//  RndMeth=Zero
  Product6 : Product  Inputs=***/  RndMeth=Zero
  Subtract2 : Sum  Inputs=+-
  kJ/kg to J/kg : Gain  Gain=1000
  h_out_h : Outport
  T_out_h : Outport  Port=2
  q_h : Outport  Port=3
  wires:
  [T_out] -> 2-D Lookup Table1/2
  [T_in] -> 2-D Lookup Table/2
  2-D Lookup Table/1 -> Subtract2/1
  2-D Lookup Table1/1 -> Subtract2/2
  2-D Lookup Table2/1 -> h_out_h/1
  Product6/1 -> Gain1/1
  Constant4/1 -> Product6/2
  [mdot_in] -> Product6/1
  Subtract2/1 -> Product6/3
  Fcn6/1 -> T_out_h/1, [T_out], 2-D Lookup Table2/2  "T_out"
  Mux4/1 -> Fcn6/1
  [e2NTU1] -> Mux4/3
  Constant/1 -> Mux4/2
  Gain1/1 -> q_h/1
  Constant2/1 -> Product6/4
  Product2/1 -> Gain3/1  "NTU"
  Constant9/1 -> Product2/2
  [alpha] -> Product2/1
  Constant8/1 -> Product2/3
  HTC Calc/1(alpha_a) -> [alpha]
  [T_in] -> HTC Calc/3(T_a)
  Constant10/1 -> HTC Calc/2(A_ca)
  [mdot_in] -> HTC Calc/1(mdot_a)
  [T_in] -> 2-D Lookup Table3/2
  2-D Lookup Table3/1 -> kJ/kg to J/kg/1
  Inputs/1 -> Bus Selector/1
  Bus Selector/1 -> [mdot_in]  "<mdot1_in>"
  Bus Selector/2 -> [T_in]  "<T1_in>"
  Bus Selector/3 -> [P_in]  "<P1_in>"
  Math Function3/1 -> [e2NTU1]
  Gain3/1 -> Math Function3/1
  [mdot_in] -> Product2/4
  [cp] -> Product2/5
  [T_in] -> Mux4/1
  [P_in] -> 2-D Lookup Table/1
  [P_in] -> 2-D Lookup Table1/1
  [P_in] -> 2-D Lookup Table2/1
  [P_in] -> 2-D Lookup Table3/1
  kJ/kg to J/kg/1 -> [cp]

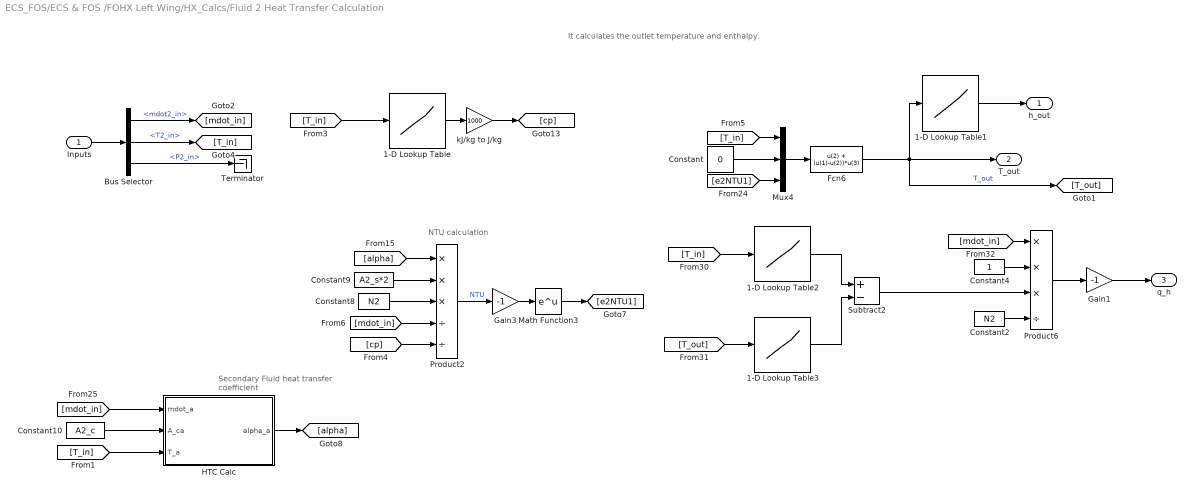
== system ECS_FOS/ECS & FOS /FOHX Left Wing/HX_Calcs/Fluid 2 Heat Transfer Calculation ==
  note: NTU calculation
  note: Secondary Fluid heat transfer coefficient
  note: It calculates the outlet temperature and enthalpy.
  Inputs : Inport
  1-D Lookup Table : Lookup_n-D  NumberOfTableDimensions=1  BreakpointsForDimension1=F2.T  Table=F2.cp_T  RndMeth=Simplest  InputSameDT=on
  1-D Lookup Table1 : Lookup_n-D  NumberOfTableDimensions=1  BreakpointsForDimension1=F2.T  Table=F2.H  RndMeth=Simplest  InputSameDT=on
  1-D Lookup Table2 : Lookup_n-D  NumberOfTableDimensions=1  BreakpointsForDimension1=F2.T  Table=F2.H  RndMeth=Simplest  InputSameDT=on
  1-D Lookup Table3 : Lookup_n-D  NumberOfTableDimensions=1  BreakpointsForDimension1=F2.T  Table=F2.H  RndMeth=Simplest  InputSameDT=on
  Bus Selector : BusSelector  OutputSignals=mdot2_in,T2_in,P2_in
  Constant : Constant  Value=0
  Constant10 : Constant  Value=A2_c
  Constant2 : Constant  Value=N2
  Constant4 : Constant
  Constant8 : Constant  Value=N2
  Constant9 : Constant  Value=A2_s*2
  Fcn6 : Fcn  Expr=u(2) + (u(1)-u(2))*u(3)
  Gain1 : Gain  Gain=-1
  Gain3 : Gain  Gain=-1
  HTC Calc : Subsystem
  Math Function3 : Math  SaturateOnIntegerOverflow=on
  Mux4 : Mux  Inputs=3
  Product2 : Product  Inputs=***//  RndMeth=Zero
  Product6 : Product  Inputs=***/  RndMeth=Zero
  Subtract2 : Sum  Inputs=+-
  Terminator : Terminator
  kJ/kg to J/kg : Gain  Gain=1000
  h_out : Outport
  T_out : Outport  Port=2
  q_h : Outport  Port=3
  wires:
  [T_out] -> 1-D Lookup Table3/1
  [T_in] -> 1-D Lookup Table2/1
  1-D Lookup Table2/1 -> Subtract2/1
  1-D Lookup Table3/1 -> Subtract2/2
  1-D Lookup Table1/1 -> h_out/1
  Product6/1 -> Gain1/1
  Constant4/1 -> Product6/2
  [mdot_in] -> Product6/1
  Subtract2/1 -> Product6/3
  Fcn6/1 -> [T_out], T_out/1, 1-D Lookup Table1/1  "T_out"
  Mux4/1 -> Fcn6/1
  [e2NTU1] -> Mux4/3
  Constant/1 -> Mux4/2
  Gain1/1 -> q_h/1
  Constant2/1 -> Product6/4
  Product2/1 -> Gain3/1  "NTU"
  Constant9/1 -> Product2/2
  [alpha] -> Product2/1
  Constant8/1 -> Product2/3
  HTC Calc/1(alpha_a) -> [alpha]
  [T_in] -> HTC Calc/3(T_a)
  Constant10/1 -> HTC Calc/2(A_ca)
  [mdot_in] -> HTC Calc/1(mdot_a)
  [T_in] -> 1-D Lookup Table/1
  1-D Lookup Table/1 -> kJ/kg to J/kg/1
  Inputs/1 -> Bus Selector/1
  Bus Selector/1 -> [mdot_in]  "<mdot2_in>"
  Bus Selector/2 -> [T_in]  "<T2_in>"
  Bus Selector/3 -> Terminator/1  "<P2_in>"
  Math Function3/1 -> [e2NTU1]
  Gain3/1 -> Math Function3/1
  [mdot_in] -> Product2/4
  [cp] -> Product2/5
  [T_in] -> Mux4/1
  kJ/kg to J/kg/1 -> [cp]

== system ECS_FOS/ECS & FOS /FOHX Left Wing/HX_Calcs/Input Processing ==
  Inputs : Inport
  Bus Creator : BusCreator  Inputs=6
  Bus Selector : BusSelector  OutputSignals=mdot1_in,P1_in,T1_in,mdot2_in,P2_in,T2_in
  Processed_Inputs : Outport
  wires:
  Bus Selector/1 -> Bus Creator/1  "<mdot1_in>"
  Bus Selector/2 -> Bus Creator/2  "<P1_in>"
  Bus Selector/3 -> Bus Creator/3  "<T1_in>"
  Bus Selector/4 -> Bus Creator/4  "<mdot2_in>"
  Bus Selector/5 -> Bus Creator/5  "<P2_in>"
  Bus Selector/6 -> Bus Creator/6  "<T2_in>"
  Inputs/1 -> Bus Selector/1  "Inputs"
  Bus Creator/1 -> Processed_Inputs/1

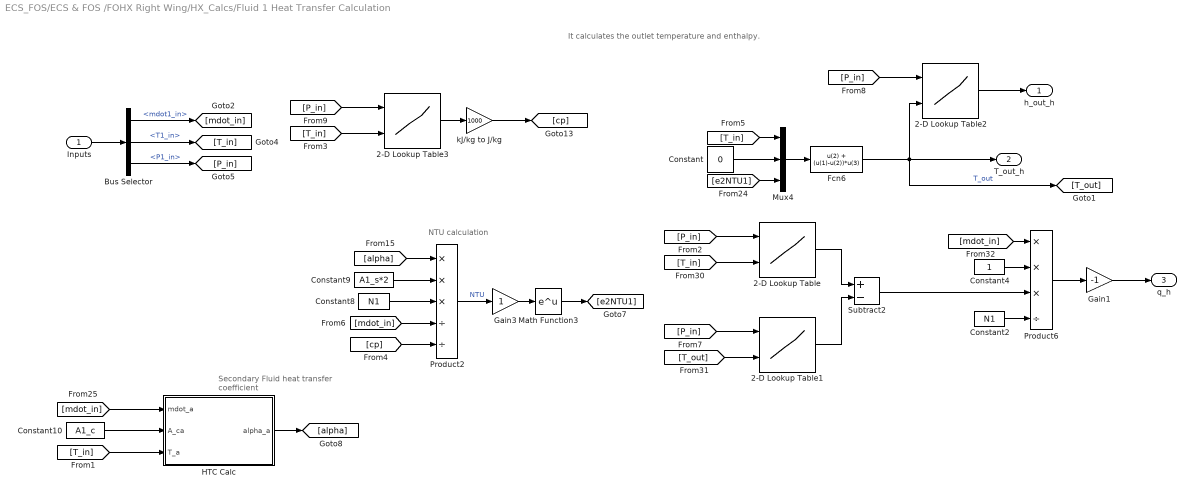
== system ECS_FOS/ECS & FOS /FOHX Right Wing/HX_Calcs/Fluid 1 Heat Transfer Calculation ==
  note: It calculates the outlet temperature and enthalpy.
  note: Secondary Fluid heat transfer coefficient
  note: NTU calculation
  Inputs : Inport
  2-D Lookup Table : Lookup_n-D  BreakpointsForDimension1=F1.P  BreakpointsForDimension2=F1.T  Table=F1.H_pt  RndMeth=Simplest  InputSameDT=on
  2-D Lookup Table1 : Lookup_n-D  BreakpointsForDimension1=F1.P  BreakpointsForDimension2=F1.T  Table=F1.H_pt  RndMeth=Simplest  InputSameDT=on
  2-D Lookup Table2 : Lookup_n-D  BreakpointsForDimension1=F1.P  BreakpointsForDimension2=F1.T  Table=F1.H_pt  RndMeth=Simplest  InputSameDT=on
  2-D Lookup Table3 : Lookup_n-D  BreakpointsForDimension1=F1.P  BreakpointsForDimension2=F1.T  Table=F1.Cp_pt  RndMeth=Simplest  InputSameDT=on
  Bus Selector : BusSelector  OutputSignals=mdot1_in,T1_in,P1_in
  Constant : Constant  Value=0
  Constant10 : Constant  Value=A1_c
  Constant2 : Constant  Value=N1
  Constant4 : Constant
  Constant8 : Constant  Value=N1
  Constant9 : Constant  Value=A1_s*2
  Fcn6 : Fcn  Expr=u(2) + (u(1)-u(2))*u(3)
  Gain1 : Gain  Gain=-1
  Gain3 : Gain
  HTC Calc : Subsystem
  Math Function3 : Math  SaturateOnIntegerOverflow=on
  Mux4 : Mux  Inputs=3
  Product2 : Product  Inputs=***//  RndMeth=Zero
  Product6 : Product  Inputs=***/  RndMeth=Zero
  Subtract2 : Sum  Inputs=+-
  kJ/kg to J/kg : Gain  Gain=1000
  h_out_h : Outport
  T_out_h : Outport  Port=2
  q_h : Outport  Port=3
  wires:
  kJ/kg to J/kg/1 -> [cp]
  [P_in] -> 2-D Lookup Table3/1
  [P_in] -> 2-D Lookup Table2/1
  [P_in] -> 2-D Lookup Table1/1
  [P_in] -> 2-D Lookup Table/1
  [T_in] -> Mux4/1
  [cp] -> Product2/5
  [mdot_in] -> Product2/4
  Gain3/1 -> Math Function3/1
  Math Function3/1 -> [e2NTU1]
  Bus Selector/3 -> [P_in]  "<P1_in>"
  Bus Selector/2 -> [T_in]  "<T1_in>"
  Bus Selector/1 -> [mdot_in]  "<mdot1_in>"
  Inputs/1 -> Bus Selector/1
  2-D Lookup Table3/1 -> kJ/kg to J/kg/1
  [T_in] -> 2-D Lookup Table3/2
  [mdot_in] -> HTC Calc/1(mdot_a)
  Constant10/1 -> HTC Calc/2(A_ca)
  [T_in] -> HTC Calc/3(T_a)
  HTC Calc/1(alpha_a) -> [alpha]
  Constant8/1 -> Product2/3
  [alpha] -> Product2/1
  Constant9/1 -> Product2/2
  Product2/1 -> Gain3/1  "NTU"
  Constant2/1 -> Product6/4
  Gain1/1 -> q_h/1
  Constant/1 -> Mux4/2
  [e2NTU1] -> Mux4/3
  Mux4/1 -> Fcn6/1
  Fcn6/1 -> 2-D Lookup Table2/2, [T_out], T_out_h/1  "T_out"
  Subtract2/1 -> Product6/3
  [mdot_in] -> Product6/1
  Constant4/1 -> Product6/2
  Product6/1 -> Gain1/1
  2-D Lookup Table2/1 -> h_out_h/1
  2-D Lookup Table1/1 -> Subtract2/2
  2-D Lookup Table/1 -> Subtract2/1
  [T_in] -> 2-D Lookup Table/2
  [T_out] -> 2-D Lookup Table1/2

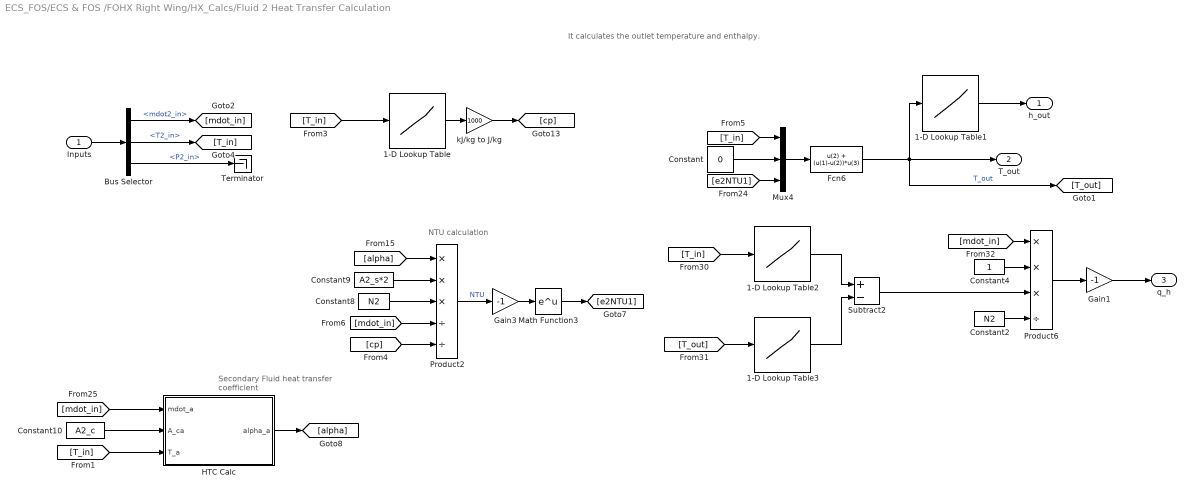
== system ECS_FOS/ECS & FOS /FOHX Right Wing/HX_Calcs/Fluid 2 Heat Transfer Calculation ==
  note: It calculates the outlet temperature and enthalpy.
  note: Secondary Fluid heat transfer coefficient
  note: NTU calculation
  Inputs : Inport
  1-D Lookup Table : Lookup_n-D  NumberOfTableDimensions=1  BreakpointsForDimension1=F2.T  Table=F2.cp_T  RndMeth=Simplest  InputSameDT=on
  1-D Lookup Table1 : Lookup_n-D  NumberOfTableDimensions=1  BreakpointsForDimension1=F2.T  Table=F2.H  RndMeth=Simplest  InputSameDT=on
  1-D Lookup Table2 : Lookup_n-D  NumberOfTableDimensions=1  BreakpointsForDimension1=F2.T  Table=F2.H  RndMeth=Simplest  InputSameDT=on
  1-D Lookup Table3 : Lookup_n-D  NumberOfTableDimensions=1  BreakpointsForDimension1=F2.T  Table=F2.H  RndMeth=Simplest  InputSameDT=on
  Bus Selector : BusSelector  OutputSignals=mdot2_in,T2_in,P2_in
  Constant : Constant  Value=0
  Constant10 : Constant  Value=A2_c
  Constant2 : Constant  Value=N2
  Constant4 : Constant
  Constant8 : Constant  Value=N2
  Constant9 : Constant  Value=A2_s*2
  Fcn6 : Fcn  Expr=u(2) + (u(1)-u(2))*u(3)
  Gain1 : Gain  Gain=-1
  Gain3 : Gain  Gain=-1
  HTC Calc : Subsystem
  Math Function3 : Math  SaturateOnIntegerOverflow=on
  Mux4 : Mux  Inputs=3
  Product2 : Product  Inputs=***//  RndMeth=Zero
  Product6 : Product  Inputs=***/  RndMeth=Zero
  Subtract2 : Sum  Inputs=+-
  Terminator : Terminator
  kJ/kg to J/kg : Gain  Gain=1000
  h_out : Outport
  T_out : Outport  Port=2
  q_h : Outport  Port=3
  wires:
  kJ/kg to J/kg/1 -> [cp]
  [T_in] -> Mux4/1
  [cp] -> Product2/5
  [mdot_in] -> Product2/4
  Gain3/1 -> Math Function3/1
  Math Function3/1 -> [e2NTU1]
  Bus Selector/3 -> Terminator/1  "<P2_in>"
  Bus Selector/2 -> [T_in]  "<T2_in>"
  Bus Selector/1 -> [mdot_in]  "<mdot2_in>"
  Inputs/1 -> Bus Selector/1
  1-D Lookup Table/1 -> kJ/kg to J/kg/1
  [T_in] -> 1-D Lookup Table/1
  [mdot_in] -> HTC Calc/1(mdot_a)
  Constant10/1 -> HTC Calc/2(A_ca)
  [T_in] -> HTC Calc/3(T_a)
  HTC Calc/1(alpha_a) -> [alpha]
  Constant8/1 -> Product2/3
  [alpha] -> Product2/1
  Constant9/1 -> Product2/2
  Product2/1 -> Gain3/1  "NTU"
  Constant2/1 -> Product6/4
  Gain1/1 -> q_h/1
  Constant/1 -> Mux4/2
  [e2NTU1] -> Mux4/3
  Mux4/1 -> Fcn6/1
  Fcn6/1 -> 1-D Lookup Table1/1, T_out/1, [T_out]  "T_out"
  Subtract2/1 -> Product6/3
  [mdot_in] -> Product6/1
  Constant4/1 -> Product6/2
  Product6/1 -> Gain1/1
  1-D Lookup Table1/1 -> h_out/1
  1-D Lookup Table3/1 -> Subtract2/2
  1-D Lookup Table2/1 -> Subtract2/1
  [T_in] -> 1-D Lookup Table2/1
  [T_out] -> 1-D Lookup Table3/1

== system ECS_FOS/ECS & FOS /FOHX Right Wing/HX_Calcs/Input Processing ==
  Inputs : Inport
  Bus Creator : BusCreator  Inputs=6
  Bus Selector : BusSelector  OutputSignals=mdot1_in,P1_in,T1_in,mdot2_in,P2_in,T2_in
  Processed_Inputs : Outport
  wires:
  Bus Creator/1 -> Processed_Inputs/1
  Inputs/1 -> Bus Selector/1  "Inputs"
  Bus Selector/6 -> Bus Creator/6  "<T2_in>"
  Bus Selector/5 -> Bus Creator/5  "<P2_in>"
  Bus Selector/4 -> Bus Creator/4  "<mdot2_in>"
  Bus Selector/3 -> Bus Creator/3  "<T1_in>"
  Bus Selector/2 -> Bus Creator/2  "<P1_in>"
  Bus Selector/1 -> Bus Creator/1  "<mdot1_in>"

== system ECS_FOS/ECS & FOS /FOHX Left Wing/HX_Calcs/Fluid 1 Heat Transfer Calculation/HTC Calc ==
  note: Calculation of secondary fluid heat transfer coefficient using the Longo correlation
  mdot_a : Inport
  A_ca : Inport  Port=2
  T_a : Inport  Port=3
  Constant1 : Constant  Value=alpha1
  Terminator : Terminator
  Terminator1 : Terminator
  Terminator2 : Terminator
  alpha_a : Outport
  wires:
  Constant1/1 -> alpha_a/1
  mdot_a/1 -> Terminator/1
  A_ca/1 -> Terminator1/1
  T_a/1 -> Terminator2/1

== system ECS_FOS/ECS & FOS /FOHX Left Wing/HX_Calcs/Fluid 2 Heat Transfer Calculation/HTC Calc ==
  note: Calculation of secondary fluid heat transfer coefficient using the Longo correlation
  mdot_a : Inport
  A_ca : Inport  Port=2
  T_a : Inport  Port=3
  Constant1 : Constant  Value=alpha2
  Terminator : Terminator
  Terminator1 : Terminator
  Terminator2 : Terminator
  alpha_a : Outport
  wires:
  Constant1/1 -> alpha_a/1
  mdot_a/1 -> Terminator/1
  A_ca/1 -> Terminator1/1
  T_a/1 -> Terminator2/1

== system ECS_FOS/ECS & FOS /FOHX Right Wing/HX_Calcs/Fluid 1 Heat Transfer Calculation/HTC Calc ==
  note: Calculation of secondary fluid heat transfer coefficient using the Longo correlation
  mdot_a : Inport
  A_ca : Inport  Port=2
  T_a : Inport  Port=3
  Constant1 : Constant  Value=alpha1
  Terminator : Terminator
  Terminator1 : Terminator
  Terminator2 : Terminator
  alpha_a : Outport
  wires:
  T_a/1 -> Terminator2/1
  A_ca/1 -> Terminator1/1
  mdot_a/1 -> Terminator/1
  Constant1/1 -> alpha_a/1

== system ECS_FOS/ECS & FOS /FOHX Right Wing/HX_Calcs/Fluid 2 Heat Transfer Calculation/HTC Calc ==
  note: Calculation of secondary fluid heat transfer coefficient using the Longo correlation
  mdot_a : Inport
  A_ca : Inport  Port=2
  T_a : Inport  Port=3
  Constant1 : Constant  Value=alpha2
  Terminator : Terminator
  Terminator1 : Terminator
  Terminator2 : Terminator
  alpha_a : Outport
  wires:
  T_a/1 -> Terminator2/1
  A_ca/1 -> Terminator1/1
  mdot_a/1 -> Terminator/1
  Constant1/1 -> alpha_a/1
